simulink model "q7_LQR_based_data_set_sim"  (R2019a)
settings: Solver=VariableStepAuto  StartTime=0.0  StopTime=T  RelTol=1e-3
values from neighbouring files (symbols this model uses):
  A = bsxfun(@rdivide, A, diag(A))    [Q7_LQR_Based_Data_Without_Simulink.m]
  B = [B1, B2]    [Q7_LQR_Based_Data_Without_Simulink.m]
  C = [0 0 1 0 0 0]    [Q7_LQR_Based_Data_Without_Simulink.m]
  k_sim = K_ADP    [Q7_LQR_Based_Data_Without_Simulink.m]
  Ts = 0.01    [Q7_LQR_Based_Data_Without_Simulink.m]
  x0 = [0;0;0;0;0;0]    [Q7_LQR_Based_Data_Without_Simulink.m]
settings Model: Creator=ronil  LastModifiedBy=ronil

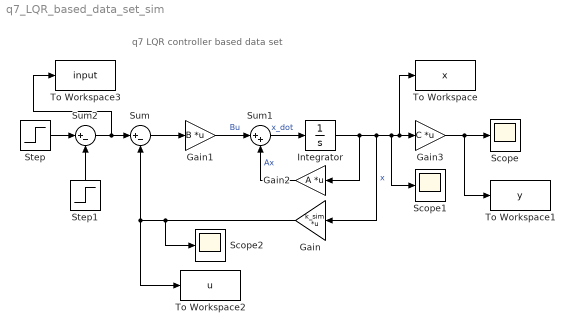
== system q7_LQR_based_data_set_sim ==
  note: q7 LQR controller based data set
  Gain : Gain  Gain=k_sim  Multiplication=Matrix(K*u)
  Gain1 : Gain  Gain=B  Multiplication=Matrix(K*u)
  Gain2 : Gain  Gain=A  Multiplication=Matrix(K*u)
  Gain3 : Gain  Gain=C  Multiplication=Matrix(K*u)
  Integrator : Integrator  InitialCondition=x0
  Scope : Scope
  Scope1 : Scope
  Scope2 : Scope
  Step : Step  After=50  SampleTime=Ts
  Step1 : Step  Time=1.5  After=50  SampleTime=Ts
  Sum : Sum  Inputs=|+-
  Sum1 : Sum  Inputs=|++
  Sum2 : Sum  Inputs=|+-
  To Workspace : ToWorkspace  VariableName=x  SaveFormat=Timeseries  SampleTime=Ts
  To Workspace1 : ToWorkspace  VariableName=y  SaveFormat=Timeseries  SampleTime=-1
  To Workspace2 : ToWorkspace  VariableName=u  SaveFormat=Timeseries  SampleTime=-1
  To Workspace3 : ToWorkspace  VariableName=input  SaveFormat=Timeseries  SampleTime=-1
  wires:
  Gain1/1 -> Sum1/1  "Bu"
  Gain2/1 -> Sum1/2  "Ax"
  Gain/1 -> Sum/2, To Workspace2/1, Scope2/1
  Integrator/1 -> Gain/1, Scope1/1, To Workspace/1, Gain3/1, Gain2/1  "x"
  Gain3/1 -> To Workspace1/1, Scope/1
  Sum1/1 -> Integrator/1  "x_dot"
  Sum/1 -> Gain1/1
  Step1/1 -> Sum2/2
  Step/1 -> Sum2/1
  Sum2/1 -> To Workspace3/1, Sum/1
